simulink model "power_wind_dfig"  (R2023a)
settings: Solver=ode23tb  StartTime=0.0  StopTime=50  MaxStep=1/60  RelTol=1e-4  AbsTol=1e-3  EnableMultiTasking=on
InitFcn:
  | xInitial = init_power_wind_dfig;
undefined symbols (not defined in the file): D1, D11, Delta, F, find_system, Fnom, gcbh, H, ILd_init, ILq_init, Imax_grid_conv, Init, j, Ki_dc_reg, Ki_grid_side_cur_reg, Ki_power_reg, Ki_Q, Ki_rotor_side_cur_reg, Ki_volt_reg, Kp_dc_reg, Kp_grid_side_cur_reg, Kp_power_reg, Kp_Q, Kp_rotor_side_cur_reg, Kp_volt_reg, L_RL, Llr, Lls, p, Pnom, power_A, power_B, power_D, R_RL, Rr, Rs, speed_A, speed_B, speed_C, speed_D, sps_rtmsupport, Vcontrol, Vnom, Wind_On
libraries: spsOnDelayLib x18, spsThreePhaseVIMeasurementLib x6, simulink_extras x5, spsThreePhaseTransformerTwoWindingsLib x4, spsControlledCurrentSourceLib x4, spsGroundLib x3, spsThreePhaseSeriesRLCLoadLib x3, spsPower3phPhasorLib x3, spsBistableLib x3, spsThreePhasePISectionLineLib x2, spsSeriesRLCBranchLib x2, spsSequenceAnalyzerPhasorLib x2
(part 3 of 6)

== system power_wind_dfig/Measurements/Wind turbine Data acquisition/magnitude positive seq. /Fourier1 ==
  signal : Inport
  Constant : Constant  Value=0
  Fcn : Fcn  Expr=u^2
  Fcn1 : Fcn  Expr=u^2
  Fcn2 : Fcn  Expr=sqrt(u)
  Fcn3 : Fcn  Expr=180/pi*atan2(u[2],u[1])
  Gain1 : Gain  Gain=k*f1  SaturateOnIntegerOverflow=on  OutDataTypeStr=Inherit: Same as input  ParamDataTypeStr=Inherit: Same as input
  Integ2 : Integrator  InitialConditionSource=external
  Mux : Mux  Inputs=2
  Product : Product  InputSameDT=on  SaturateOnIntegerOverflow=on  OutDataTypeStr=Inherit: Same as first input
  Product1 : Product  InputSameDT=on  SaturateOnIntegerOverflow=on  OutDataTypeStr=Inherit: Same as first input
  Sum : Sum  InputSameDT=on  SaturateOnIntegerOverflow=on  OutDataTypeStr=Inherit: Same as first input
  Sum1 : Sum  Inputs=+-  InputSameDT=on  SaturateOnIntegerOverflow=on  OutDataTypeStr=Inherit: Same as first input
  Sum2 : Sum  Inputs=+-  InputSameDT=on  SaturateOnIntegerOverflow=on  OutDataTypeStr=Inherit: Same as first input
  T : TransportDelay  DelayTime=1/f1  BufferSize=2048
  T1 : TransportDelay  DelayTime=1/f1  BufferSize=2048
  cos(nwt) : Sin  Frequency=2*pi*n*f1  Phase=pi/2  SampleTime=0
  integ1 : Integrator  InitialConditionSource=external
  sin(nwt) : Sin  Frequency=2*pi*n*f1  SampleTime=0
  magnitude : Outport  InitialOutput=0  VectorParamsAs1DForOutWhenUnconnected=off
  angle : Outport  Port=2  InitialOutput=0  VectorParamsAs1DForOutWhenUnconnected=off
  wires:
  Constant/1 -> integ1/2, Integ2/2
  Sum/1 -> Fcn2/1
  Fcn/1 -> Sum/1
  Fcn1/1 -> Sum/2
  Mux/1 -> Fcn3/1
  Fcn3/1 -> angle/1
  sin(nwt)/1 -> Product/1
  cos(nwt)/1 -> Product1/2
  Product/1 -> integ1/1
  Product1/1 -> Integ2/1
  T/1 -> Sum1/2
  T1/1 -> Sum2/2
  integ1/1 -> Sum1/1, T/1
  Integ2/1 -> T1/1, Sum2/1
  Sum2/1 -> Fcn1/1, Mux/2
  Sum1/1 -> Fcn/1, Mux/1
  signal/1 -> Gain1/1
  Gain1/1 -> Product/2, Product1/1
  Fcn2/1 -> magnitude/1

== system power_wind_dfig/Measurements/Wind turbine Data acquisition/magnitude positive seq. /Fourier2 ==
  signal : Inport
  Constant : Constant  Value=0
  Fcn : Fcn  Expr=u^2
  Fcn1 : Fcn  Expr=u^2
  Fcn2 : Fcn  Expr=sqrt(u)
  Fcn3 : Fcn  Expr=180/pi*atan2(u[2],u[1])
  Gain1 : Gain  Gain=k*f1  SaturateOnIntegerOverflow=on  OutDataTypeStr=Inherit: Same as input  ParamDataTypeStr=Inherit: Same as input
  Integ2 : Integrator  InitialConditionSource=external
  Mux : Mux  Inputs=2
  Product : Product  InputSameDT=on  SaturateOnIntegerOverflow=on  OutDataTypeStr=Inherit: Same as first input
  Product1 : Product  InputSameDT=on  SaturateOnIntegerOverflow=on  OutDataTypeStr=Inherit: Same as first input
  Sum : Sum  InputSameDT=on  SaturateOnIntegerOverflow=on  OutDataTypeStr=Inherit: Same as first input
  Sum1 : Sum  Inputs=+-  InputSameDT=on  SaturateOnIntegerOverflow=on  OutDataTypeStr=Inherit: Same as first input
  Sum2 : Sum  Inputs=+-  InputSameDT=on  SaturateOnIntegerOverflow=on  OutDataTypeStr=Inherit: Same as first input
  T : TransportDelay  DelayTime=1/f1  BufferSize=2048
  T1 : TransportDelay  DelayTime=1/f1  BufferSize=2048
  cos(nwt) : Sin  Frequency=2*pi*n*f1  Phase=pi/2  SampleTime=0
  integ1 : Integrator  InitialConditionSource=external
  sin(nwt) : Sin  Frequency=2*pi*n*f1  SampleTime=0
  magnitude : Outport  InitialOutput=0  VectorParamsAs1DForOutWhenUnconnected=off
  angle : Outport  Port=2  InitialOutput=0  VectorParamsAs1DForOutWhenUnconnected=off
  wires:
  Fcn2/1 -> magnitude/1
  Gain1/1 -> Product1/1, Product/2
  signal/1 -> Gain1/1
  Sum1/1 -> Mux/1, Fcn/1
  Sum2/1 -> Mux/2, Fcn1/1
  Integ2/1 -> Sum2/1, T1/1
  integ1/1 -> T/1, Sum1/1
  T1/1 -> Sum2/2
  T/1 -> Sum1/2
  Product1/1 -> Integ2/1
  Product/1 -> integ1/1
  cos(nwt)/1 -> Product1/2
  sin(nwt)/1 -> Product/1
  Fcn3/1 -> angle/1
  Mux/1 -> Fcn3/1
  Fcn1/1 -> Sum/2
  Fcn/1 -> Sum/1
  Sum/1 -> Fcn2/1
  Constant/1 -> Integ2/2, integ1/2

== system power_wind_dfig/Measurements/Wind turbine Data acquisition/magnitude positivie seq/Fourier1 ==
  signal : Inport
  Constant : Constant  Value=0
  Fcn : Fcn  Expr=u^2
  Fcn1 : Fcn  Expr=u^2
  Fcn2 : Fcn  Expr=sqrt(u)
  Fcn3 : Fcn  Expr=180/pi*atan2(u[2],u[1])
  Gain1 : Gain  Gain=k*f1  SaturateOnIntegerOverflow=on  OutDataTypeStr=Inherit: Same as input  ParamDataTypeStr=Inherit: Same as input
  Integ2 : Integrator  InitialConditionSource=external
  Mux : Mux  Inputs=2
  Product : Product  InputSameDT=on  SaturateOnIntegerOverflow=on  OutDataTypeStr=Inherit: Same as first input
  Product1 : Product  InputSameDT=on  SaturateOnIntegerOverflow=on  OutDataTypeStr=Inherit: Same as first input
  Sum : Sum  InputSameDT=on  SaturateOnIntegerOverflow=on  OutDataTypeStr=Inherit: Same as first input
  Sum1 : Sum  Inputs=+-  InputSameDT=on  SaturateOnIntegerOverflow=on  OutDataTypeStr=Inherit: Same as first input
  Sum2 : Sum  Inputs=+-  InputSameDT=on  SaturateOnIntegerOverflow=on  OutDataTypeStr=Inherit: Same as first input
  T : TransportDelay  DelayTime=1/f1  BufferSize=2048
  T1 : TransportDelay  DelayTime=1/f1  BufferSize=2048
  cos(nwt) : Sin  Frequency=2*pi*n*f1  Phase=pi/2  SampleTime=0
  integ1 : Integrator  InitialConditionSource=external
  sin(nwt) : Sin  Frequency=2*pi*n*f1  SampleTime=0
  magnitude : Outport  InitialOutput=0  VectorParamsAs1DForOutWhenUnconnected=off
  angle : Outport  Port=2  InitialOutput=0  VectorParamsAs1DForOutWhenUnconnected=off
  wires:
  Fcn2/1 -> magnitude/1
  Gain1/1 -> Product1/1, Product/2
  signal/1 -> Gain1/1
  Sum1/1 -> Mux/1, Fcn/1
  Sum2/1 -> Mux/2, Fcn1/1
  Integ2/1 -> Sum2/1, T1/1
  integ1/1 -> T/1, Sum1/1
  T1/1 -> Sum2/2
  T/1 -> Sum1/2
  Product1/1 -> Integ2/1
  Product/1 -> integ1/1
  cos(nwt)/1 -> Product1/2
  sin(nwt)/1 -> Product/1
  Fcn3/1 -> angle/1
  Mux/1 -> Fcn3/1
  Fcn1/1 -> Sum/2
  Fcn/1 -> Sum/1
  Sum/1 -> Fcn2/1
  Constant/1 -> Integ2/2, integ1/2

== system power_wind_dfig/Measurements/Wind turbine Data acquisition/magnitude positivie seq/Fourier2 ==
  signal : Inport
  Constant : Constant  Value=0
  Fcn : Fcn  Expr=u^2
  Fcn1 : Fcn  Expr=u^2
  Fcn2 : Fcn  Expr=sqrt(u)
  Fcn3 : Fcn  Expr=180/pi*atan2(u[2],u[1])
  Gain1 : Gain  Gain=k*f1  SaturateOnIntegerOverflow=on  OutDataTypeStr=Inherit: Same as input  ParamDataTypeStr=Inherit: Same as input
  Integ2 : Integrator  InitialConditionSource=external
  Mux : Mux  Inputs=2
  Product : Product  InputSameDT=on  SaturateOnIntegerOverflow=on  OutDataTypeStr=Inherit: Same as first input
  Product1 : Product  InputSameDT=on  SaturateOnIntegerOverflow=on  OutDataTypeStr=Inherit: Same as first input
  Sum : Sum  InputSameDT=on  SaturateOnIntegerOverflow=on  OutDataTypeStr=Inherit: Same as first input
  Sum1 : Sum  Inputs=+-  InputSameDT=on  SaturateOnIntegerOverflow=on  OutDataTypeStr=Inherit: Same as first input
  Sum2 : Sum  Inputs=+-  InputSameDT=on  SaturateOnIntegerOverflow=on  OutDataTypeStr=Inherit: Same as first input
  T : TransportDelay  DelayTime=1/f1  BufferSize=2048
  T1 : TransportDelay  DelayTime=1/f1  BufferSize=2048
  cos(nwt) : Sin  Frequency=2*pi*n*f1  Phase=pi/2  SampleTime=0
  integ1 : Integrator  InitialConditionSource=external
  sin(nwt) : Sin  Frequency=2*pi*n*f1  SampleTime=0
  magnitude : Outport  InitialOutput=0  VectorParamsAs1DForOutWhenUnconnected=off
  angle : Outport  Port=2  InitialOutput=0  VectorParamsAs1DForOutWhenUnconnected=off
  wires:
  Constant/1 -> integ1/2, Integ2/2
  Sum/1 -> Fcn2/1
  Fcn/1 -> Sum/1
  Fcn1/1 -> Sum/2
  Mux/1 -> Fcn3/1
  Fcn3/1 -> angle/1
  sin(nwt)/1 -> Product/1
  cos(nwt)/1 -> Product1/2
  Product/1 -> integ1/1
  Product1/1 -> Integ2/1
  T/1 -> Sum1/2
  T1/1 -> Sum2/2
  integ1/1 -> Sum1/1, T/1
  Integ2/1 -> T1/1, Sum2/1
  Sum2/1 -> Fcn1/1, Mux/2
  Sum1/1 -> Fcn/1, Mux/1
  signal/1 -> Gain1/1
  Gain1/1 -> Product/2, Product1/1
  Fcn2/1 -> magnitude/1

== system power_wind_dfig/Plant 2 MVA/Plant & Motor Protection/AC Current Protection/Current Measurement ==
  abc : Inport  PortDimensions=3
  Gain1 : Gain  Gain=[1 a a2]  SaturateOnIntegerOverflow=on  OutDataTypeStr=Inherit: Same as input  ParamDataTypeStr=Inherit: Same as input
  Gain2 : Gain  Gain=[1 a2 a]  SaturateOnIntegerOverflow=on  OutDataTypeStr=Inherit: Same as input  ParamDataTypeStr=Inherit: Same as input
  Gain3 : Gain  Gain=1/3  SaturateOnIntegerOverflow=on  OutDataTypeStr=Inherit: Same as input  ParamDataTypeStr=Inherit: Same as input
  Gain4 : Gain  Gain=1/3  SaturateOnIntegerOverflow=on  OutDataTypeStr=Inherit: Same as input  ParamDataTypeStr=Inherit: Same as input
  Mux : Mux  Inputs=3
  Product : Product  Inputs=/*  SaturateOnIntegerOverflow=on  OutDataTypeStr=Inherit: Same as first input
  Saturation : Saturate  UpperLimit=1e6  LowerLimit=1e-6
  Selector : Selector  InputPortWidth=3  IndexOptions=Index vector (dialog)  Indices=1  OutputSizes=1
  Selector1 : Selector  InputPortWidth=3  IndexOptions=Index vector (dialog)  Indices=2  OutputSizes=1
  Selector2 : Selector  InputPortWidth=3  IndexOptions=Index vector (dialog)  Indices=3  OutputSizes=1
  Sum : Sum  Inputs=1  InputSameDT=on  SaturateOnIntegerOverflow=on  OutDataTypeStr=Inherit: Same as first input
  Sum1 : Sum  Inputs=1  InputSameDT=on  SaturateOnIntegerOverflow=on  OutDataTypeStr=Inherit: Same as first input
  magnitude : Subsystem
  magnitude1 : Subsystem
  I1 : Outport  VectorParamsAs1DForOutWhenUnconnected=off
  I2/I1 : Outport  Port=2  VectorParamsAs1DForOutWhenUnconnected=off
  wires:
  magnitude/1(Out1) -> I1/1, Saturation/1
  magnitude1/1(Out1) -> Product/2
  Product/1 -> I2/I1/1
  Saturation/1 -> Product/1
  Gain4/1 -> magnitude1/1(In1)
  Gain3/1 -> magnitude/1(In1)
  Mux/1 -> Gain2/1, Gain1/1
  abc/1 -> Selector/1, Selector1/1, Selector2/1
  Gain2/1 -> Sum1/1
  Sum1/1 -> Gain4/1
  Gain1/1 -> Sum/1
  Sum/1 -> Gain3/1
  Selector/1 -> Mux/1
  Selector1/1 -> Mux/2
  Selector2/1 -> Mux/3

== system power_wind_dfig/Plant 2 MVA/Plant & Motor Protection/AC Voltage Protection/Voltage Measurement ==
  abc : Inport  PortDimensions=3
  Gain1 : Gain  Gain=[1 a a2]  SaturateOnIntegerOverflow=on  OutDataTypeStr=Inherit: Same as input  ParamDataTypeStr=Inherit: Same as input
  Gain2 : Gain  Gain=[1 a2 a]  SaturateOnIntegerOverflow=on  OutDataTypeStr=Inherit: Same as input  ParamDataTypeStr=Inherit: Same as input
  Gain3 : Gain  Gain=1/3  SaturateOnIntegerOverflow=on  OutDataTypeStr=Inherit: Same as input  ParamDataTypeStr=Inherit: Same as input
  Gain4 : Gain  Gain=1/3  SaturateOnIntegerOverflow=on  OutDataTypeStr=Inherit: Same as input  ParamDataTypeStr=Inherit: Same as input
  Gain5 : Gain  Gain=1/3  SaturateOnIntegerOverflow=on  OutDataTypeStr=Inherit: Same as input  ParamDataTypeStr=Inherit: Same as input
  Mux : Mux  Inputs=3
  Product : Product  Inputs=/*  SaturateOnIntegerOverflow=on  OutDataTypeStr=Inherit: Same as first input
  Product1 : Product  Inputs=/*  SaturateOnIntegerOverflow=on  OutDataTypeStr=Inherit: Same as first input
  Saturation : Saturate  UpperLimit=1e6  LowerLimit=1e-6
  Selector : Selector  InputPortWidth=3  IndexOptions=Index vector (dialog)  Indices=1  OutputSizes=1
  Selector1 : Selector  InputPortWidth=3  IndexOptions=Index vector (dialog)  Indices=2  OutputSizes=1
  Selector2 : Selector  InputPortWidth=3  IndexOptions=Index vector (dialog)  Indices=3  OutputSizes=1
  Sum : Sum  Inputs=1  InputSameDT=on  SaturateOnIntegerOverflow=on  OutDataTypeStr=Inherit: Same as first input
  Sum1 : Sum  Inputs=1  InputSameDT=on  SaturateOnIntegerOverflow=on  OutDataTypeStr=Inherit: Same as first input
  Sum2 : Sum  Inputs=1  InputSameDT=on  SaturateOnIntegerOverflow=on  OutDataTypeStr=Inherit: Same as first input
  magnitude : Subsystem
  magnitude1 : Subsystem
  magnitude2 : Subsystem
  V1 : Outport  VectorParamsAs1DForOutWhenUnconnected=off
  V2/V1 : Outport  Port=2  VectorParamsAs1DForOutWhenUnconnected=off
  V0/V1 : Outport  Port=3  VectorParamsAs1DForOutWhenUnconnected=off
  wires:
  magnitude2/1(Out1) -> Product1/2
  magnitude1/1(Out1) -> Product/2
  magnitude/1(Out1) -> Saturation/1, V1/1
  Sum/1 -> Gain3/1
  Gain1/1 -> Sum/1
  Sum1/1 -> Gain4/1
  Gain2/1 -> Sum1/1
  Sum2/1 -> Gain5/1
  Mux/1 -> Gain1/1, Gain2/1, Sum2/1
  Gain3/1 -> magnitude/1(In1)
  Gain4/1 -> magnitude1/1(In1)
  Saturation/1 -> Product/1, Product1/1
  Gain5/1 -> magnitude2/1(In1)
  Product/1 -> V2/V1/1
  Product1/1 -> V0/V1/1
  abc/1 -> Selector/1, Selector1/1, Selector2/1
  Selector/1 -> Mux/1
  Selector1/1 -> Mux/2
  Selector2/1 -> Mux/3

== system power_wind_dfig/Wind Turbine Doubly-Fed Induction Generator (Phasor Type)/Generator & Converters/Asynchronous machine Positive sequence phasor model Inputs and outputs are in per unit (pu)/Mechanical ==
  Tm : Inport
  phiqds1,iqds1 : Inport  Port=2
  1\p : Gain  Gain=1/p  SaturateOnIntegerOverflow=on  OutDataTypeStr=Inherit: Same as input  ParamDataTypeStr=Inherit: Same as input
  1_2H : Gain  Gain=1/(2*H)  SaturateOnIntegerOverflow=on  OutDataTypeStr=Inherit: Same as input  ParamDataTypeStr=Inherit: Same as input
  F : Gain  Gain=F  SaturateOnIntegerOverflow=on  OutDataTypeStr=Inherit: Same as input  ParamDataTypeStr=Inherit: Same as input
  Integrator : Integrator  InitialCondition=wmo  LowerSaturationLimit=0
  Integrator1 : Integrator  InitialCondition=tho
  Mux4 : Mux  Inputs=3
  Product1 : Product  Inputs=1  InputSameDT=on  SaturateOnIntegerOverflow=on  OutDataTypeStr=Inherit: Same as first input
  Product2 : Product  Inputs=1  InputSameDT=on  SaturateOnIntegerOverflow=on  OutDataTypeStr=Inherit: Same as first input
  Selector : Selector  InputPortWidth=4  IndexOptions=Index vector (dialog)  Indices=[1 4]  OutputSizes=1
  Selector1 : Selector  InputPortWidth=4  IndexOptions=Index vector (dialog)  Indices=[2 3]  OutputSizes=1
  Sum : Sum  Inputs=-+-  InputSameDT=on  SaturateOnIntegerOverflow=on  OutDataTypeStr=Inherit: Same as first input
  Sum1 : Sum  Inputs=|-+  InputSameDT=on  SaturateOnIntegerOverflow=on  OutDataTypeStr=Inherit: Same as first input
  web : Gain  Gain=web  SaturateOnIntegerOverflow=on  OutDataTypeStr=Inherit: Same as input  ParamDataTypeStr=Inherit: Same as input
  wr,Te,thr : Outport  VectorParamsAs1DForOutWhenUnconnected=off
  wires:
  Sum1/1 -> Sum/2, Mux4/2  "Pos.seq.Torque"
  Integrator1/1 -> 1\p/1
  1\p/1 -> Mux4/3
  web/1 -> Integrator1/1
  F/1 -> Sum/3
  Integrator/1 -> web/1, Mux4/1, F/1  "w (pu)"
  1_2H/1 -> Integrator/1
  Sum/1 -> 1_2H/1
  Tm/1 -> Sum/1  "Tm"
  Mux4/1 -> wr,Te,thr/1
  Product1/1 -> Sum1/1
  Product2/1 -> Sum1/2
  phiqds1,iqds1/1 -> Selector/1, Selector1/1
  Selector1/1 -> Product2/1
  Selector/1 -> Product1/1

== system power_wind_dfig/Wind Turbine Doubly-Fed Induction Generator (Phasor Type)/Generator & Converters/Asynchronous machine Positive sequence phasor model Inputs and outputs are in per unit (pu)/Phasors Ia Ib stator ==
  note: Ia= I1
  note: Ib= a^2*I1
  note: I1
  Idqs1 : Inport
  Demux : Demux  Outputs=2
      settings: DisplayOption=none
  Mux1 : Mux  Inputs=2
  Mux2 : Mux  Inputs=[2 1]
  Real-Imag to Complex : RealImagToComplex
  Sum : Sum  Inputs=1  InputSameDT=on  SaturateOnIntegerOverflow=on  OutDataTypeStr=Inherit: Same as first input
  a^2 : Gain  Gain=exp(-j*2*pi/3)  SaturateOnIntegerOverflow=on  OutDataTypeStr=Inherit: Same as input  ParamDataTypeStr=Inherit: Same as input
  inv : Gain  Gain=-1  SaturateOnIntegerOverflow=on  OutDataTypeStr=Inherit: Same as input  ParamDataTypeStr=Inherit: Same as input
  Isabc cmplx : Outport  VectorParamsAs1DForOutWhenUnconnected=off
  wires:
  Demux/2 -> Real-Imag to Complex/2
  Demux/1 -> Real-Imag to Complex/1
  a^2/1 -> Mux1/2
  Idqs1/1 -> Demux/1
  Mux1/1 -> Mux2/1, Sum/1  "ia ib"
  Sum/1 -> inv/1
  inv/1 -> Mux2/2  "ic"
  Mux2/1 -> Isabc cmplx/1
  Real-Imag to Complex/1 -> Mux1/1, a^2/1  "I1"

== system power_wind_dfig/Wind Turbine Doubly-Fed Induction Generator (Phasor Type)/Generator & Converters/Asynchronous machine Positive sequence phasor model Inputs and outputs are in per unit (pu)/Positive Sequence Model ==
  Vqdr1 : Inport
  w-wr : Inport  Port=2
  Vqds1 : Inport  Port=3
  Trip : Inport  Port=4
  Constant7 : Constant
  Mutual fluxes : Subsystem
  Rotor : Subsystem
      mask Display: disp('Rotor')
  Stator : Subsystem
      mask Display: disp('Stator')
  Iqdr1 : Outport  VectorParamsAs1DForOutWhenUnconnected=off
  Iqds1 : Outport  Port=2  VectorParamsAs1DForOutWhenUnconnected=off
  Phiqds1_Isqds1 : Outport  Port=3  VectorParamsAs1DForOutWhenUnconnected=off
  wires:
  Stator/3(phis,is) -> Phiqds1_Isqds1/1
  Stator/2(iqs,ids) -> Iqds1/1
  w-wr/1 -> Rotor/2(w-wr)
  Rotor/1(iqr,idr) -> Iqdr1/1
  Vqds1/1 -> Stator/2(vqs,vds)
  Vqdr1/1 -> Rotor/1(vqr,vdr)
  Constant7/1 -> Stator/3(w)
  Rotor/2(phiqr,phidr) -> Mutual fluxes/1(phiqr,phidr)
  Stator/1(phiqs,phids) -> Mutual fluxes/2(phiqs,phids)
  Mutual fluxes/1(phimq,phimd) -> Stator/1(phimq,phimd), Rotor/3(phimq,phimd)
  Trip/1 -> Stator/4(Trip), Rotor/4(Trip)

== system power_wind_dfig/Wind Turbine Doubly-Fed Induction Generator (Phasor Type)/Generator & Converters/Asynchronous machine Positive sequence phasor model Inputs and outputs are in per unit (pu)/Vab Vbc ==
  Vabc : Inport
  Mux : Mux  Inputs=2
  Selector : Selector  InputPortWidth=3  IndexOptions=Index vector (dialog)  Indices=[1]  OutputSizes=1
  Selector1 : Selector  InputPortWidth=3  IndexOptions=Index vector (dialog)  Indices=[2]  OutputSizes=1
  Selector2 : Selector  InputPortWidth=3  IndexOptions=Index vector (dialog)  Indices=[3]  OutputSizes=1
  Sum : Sum  Inputs=|+-  SaturateOnIntegerOverflow=on
  Sum1 : Sum  Inputs=|+-  SaturateOnIntegerOverflow=on
  Vab_Vbc : Outport  VectorParamsAs1DForOutWhenUnconnected=off
  wires:
  Vabc/1 -> Selector2/1, Selector1/1, Selector/1
  Selector/1 -> Sum/1  "Va"
  Selector1/1 -> Sum/2, Sum1/1  "Vb"
  Sum/1 -> Mux/1  "Vab"
  Selector2/1 -> Sum1/2  "Vc"
  Sum1/1 -> Mux/2  "Vbc"
  Mux/1 -> Vab_Vbc/1

== system power_wind_dfig/Wind Turbine Doubly-Fed Induction Generator (Phasor Type)/Generator & Converters/Asynchronous machine Positive sequence phasor model Inputs and outputs are in per unit (pu)/abc2dq ==
  note: V1= 1/3(Vab -a^2*Vbc)
  Vab Vbc cmplx : Inport
  (a^2)/3 : Gain  Gain=1/3*exp(-j*2*pi/3)  SaturateOnIntegerOverflow=on  OutDataTypeStr=Inherit: Same as input  ParamDataTypeStr=Inherit: Same as input
  Complex to Real-Imag : ComplexToRealImag
  Demux : Demux  Outputs=2
      settings: DisplayOption=none
  Gain : Gain  Gain=1/3  SaturateOnIntegerOverflow=on  OutDataTypeStr=Inherit: Same as input  ParamDataTypeStr=Inherit: Same as input
  Mux : Mux  Inputs=2
  Sum3 : Sum  Inputs=+-  InputSameDT=on  SaturateOnIntegerOverflow=on  OutDataTypeStr=Inherit: Same as first input
  Vdqs1 : Outport  VectorParamsAs1DForOutWhenUnconnected=off
  wires:
  Complex to Real-Imag/2 -> Mux/2  "Vq_stator (pu)"
  Complex to Real-Imag/1 -> Mux/1  "Vd_stator (pu)"
  Mux/1 -> Vdqs1/1
  Sum3/1 -> Complex to Real-Imag/1  "V1"
  Demux/1 -> Gain/1
  Vab Vbc cmplx/1 -> Demux/1
  Gain/1 -> Sum3/1
  (a^2)/3/1 -> Sum3/2
  Demux/2 -> (a^2)/3/1

== system power_wind_dfig/Wind Turbine Doubly-Fed Induction Generator (Phasor Type)/Generator & Converters/Control/Converters voltages ==
  Vdq_ctrl_grid_conv : Inport
  Vdc : Inport  Port=2
  Vdq_ctrl_rotor_conv : Inport  Port=3
  ->pu : Gain  Gain=1/(Vnom*sqrt(2)/sqrt(3))  SaturateOnIntegerOverflow=on  OutDataTypeStr=Inherit: Same as input  ParamDataTypeStr=Inherit: Same as input
  "->pu " : Gain  Gain=1/(Vnom*sqrt(2)/sqrt(3))  SaturateOnIntegerOverflow=on  OutDataTypeStr=Inherit: Same as input  ParamDataTypeStr=Inherit: Same as input
  Complex to Real-Imag : ComplexToRealImag
  Complex to Real-Imag1 : ComplexToRealImag
  Gain : Gain  Gain=1/2  SaturateOnIntegerOverflow=on  OutDataTypeStr=Inherit: Same as input  ParamDataTypeStr=Inherit: Same as input
  Gain1 : Gain  Gain=1/2  SaturateOnIntegerOverflow=on  OutDataTypeStr=Inherit: Same as input  ParamDataTypeStr=Inherit: Same as input
  Mux1 : Mux  Inputs=2
  Mux2 : Mux  Inputs=2
  Product1 : Product  Inputs=**  InputSameDT=on  SaturateOnIntegerOverflow=on  OutDataTypeStr=Inherit: Same as first input
  Product2 : Product  Inputs=**  InputSameDT=on  SaturateOnIntegerOverflow=on  OutDataTypeStr=Inherit: Same as first input
  Vdq_grid_conv : Outport  VectorParamsAs1DForOutWhenUnconnected=off
  Vdq_rotor_conv : Outport  Port=2  VectorParamsAs1DForOutWhenUnconnected=off
  wires:
  Vdq_ctrl_rotor_conv/1 -> Product1/2
  Vdq_ctrl_grid_conv/1 -> Product2/1
  Product2/1 -> Gain/1
  Product1/1 -> Gain1/1
  Gain/1 -> ->pu/1
  Gain1/1 -> "->pu "/1
  Vdc/1 -> Product1/1, Product2/2
  ->pu/1 -> Complex to Real-Imag/1
  Complex to Real-Imag1/2 -> Mux2/2  "Vq_rotor (pu)"
  Mux2/1 -> Vdq_rotor_conv/1
  Complex to Real-Imag1/1 -> Mux2/1  "Vd_rotor (pu)"
  "->pu "/1 -> Complex to Real-Imag1/1
  Complex to Real-Imag/1 -> Mux1/1  "Vd_grid_conv (pu)"
  Complex to Real-Imag/2 -> Mux1/2  "Vq_grid_conv (pu)"
  Mux1/1 -> Vdq_grid_conv/1

== system power_wind_dfig/Wind Turbine Doubly-Fed Induction Generator (Phasor Type)/Generator & Converters/Control/abc2dq & Positive sequence Voltage phase angle ==
  note: V1= 1/3(Va +aVb+a^2*Vc)
  Vabc_B1 : Inport
  (a^2)/3 : Gain  Gain=1/3*exp(-j*2*pi/3)  SaturateOnIntegerOverflow=on  OutDataTypeStr=Inherit: Same as input  ParamDataTypeStr=Inherit: Same as input
  20% : Switch  Threshold=0.5  InputSameDT=off
  Complex to Magnitude-Angle : ComplexToMagnitudeAngle
  Complex to Real-Imag : ComplexToRealImag
  Demux : Demux  Outputs=3
      settings: DisplayOption=none
  Gain : Gain  Gain=1/3  SaturateOnIntegerOverflow=on  OutDataTypeStr=Inherit: Same as input  ParamDataTypeStr=Inherit: Same as input
  IC=ic : Memory  InitialCondition=-pi/2  InheritSampleTime=on
  Magnitude-Angle to Complex : MagnitudeAngleToComplex
  Mux : Mux  Inputs=2
  Relay : Relay  OnSwitchValue=0.5  OffSwitchValue=0.1
  Sum3 : Sum  Inputs=+++  InputSameDT=on  SaturateOnIntegerOverflow=on  OutDataTypeStr=Inherit: Same as first input
  a/3 : Gain  Gain=1/3*exp(j*2*pi/3)  SaturateOnIntegerOverflow=on  OutDataTypeStr=Inherit: Same as input  ParamDataTypeStr=Inherit: Same as input
  Vdq_B1 : Outport  VectorParamsAs1DForOutWhenUnconnected=off
  Theta : Outport  Port=2  VectorParamsAs1DForOutWhenUnconnected=off
  V_B1 : Outport  Port=3  VectorParamsAs1DForOutWhenUnconnected=off
  wires:
  Complex to Real-Imag/2 -> Mux/2  "Vq"
  Complex to Real-Imag/1 -> Mux/1  "Vd"
  Magnitude-Angle to Complex/1 -> Complex to Real-Imag/1
  Complex to Magnitude-Angle/1 -> Relay/1, Magnitude-Angle to Complex/1, V_B1/1
  Sum3/1 -> Complex to Magnitude-Angle/1  "V1"
  (a^2)/3/1 -> Sum3/3
  a/3/1 -> Sum3/2
  Demux/3 -> (a^2)/3/1
  Demux/2 -> a/3/1
  Gain/1 -> Sum3/1
  Vabc_B1/1 -> Demux/1
  Demux/1 -> Gain/1
  Mux/1 -> Vdq_B1/1
  20%/1 -> Theta/1, IC=ic/1
  IC=ic/1 -> 20%/3
  Relay/1 -> 20%/2
  Complex to Magnitude-Angle/2 -> Magnitude-Angle to Complex/2, 20%/1

== system power_wind_dfig/Wind Turbine Doubly-Fed Induction Generator (Phasor Type)/Generator & Converters/Control/wind_dfig_grid ==
  note: Grid-side converter control system
  Vdq_B1 : Inport
  Idq_grid_conv : Inport  Port=2
  Theta : Inport  Port=3
  Vdc : Inport  Port=4
  Iq_ref : Inport  Port=5
  Enable : EnablePort  PropagateVarSize=During execution
  Current regulator : Subsystem
  DC bus voltage Regulator : Subsystem
  Idq B1 voltage Reference frame : Subsystem
  Idq references : Subsystem
  Mux : Mux  Inputs=2
  Rate Limiter : RateLimiter  RisingSlewLimit=current_slew_rate  FallingSlewLimit=-current_slew_rate
  Subsystem : Subsystem
  Vdc_ref (V) : Constant  Value=Vdc_nom
  Vdq B1 voltage Reference frame : Subsystem
  Vdq_ctrl_grid_conv : Outport  VectorParamsAs1DForOutWhenUnconnected=off
  wires:
  Iq_ref/1 -> Rate Limiter/1
  Rate Limiter/1 -> Mux/2
  Idq references/1(Idq_ref) -> Current regulator/3(Idq_ref)
  Mux/1 -> Idq references/1(Id*Iq*)
  Idq B1 voltage Reference frame/1(Idq) -> Current regulator/2(Idq)
  DC bus voltage Regulator/1(Id_ref) -> Mux/1
  Idq_grid_conv/1 -> Idq B1 voltage Reference frame/2(Idq_grid_conv)
  Subsystem/1(Vdq_ctrl_grid_conv) -> Vdq_ctrl_grid_conv/1
  Vdc/1 -> DC bus voltage Regulator/2(Vdc), Subsystem/3(Vdc)
  Current regulator/1(Vdq*) -> Subsystem/2(Vdq*)
  Vdc_ref (V)/1 -> DC bus voltage Regulator/1(Vdc_ref)
  Theta/1 -> Subsystem/1(Theta), Vdq B1 voltage Reference frame/1(Theta), Idq B1 voltage Reference frame/1(Theta)
  Vdq_B1/1 -> Vdq B1 voltage Reference frame/2(Vdq_B1)
  Vdq B1 voltage Reference frame/1(Vdq) -> Current regulator/1(Vdq)

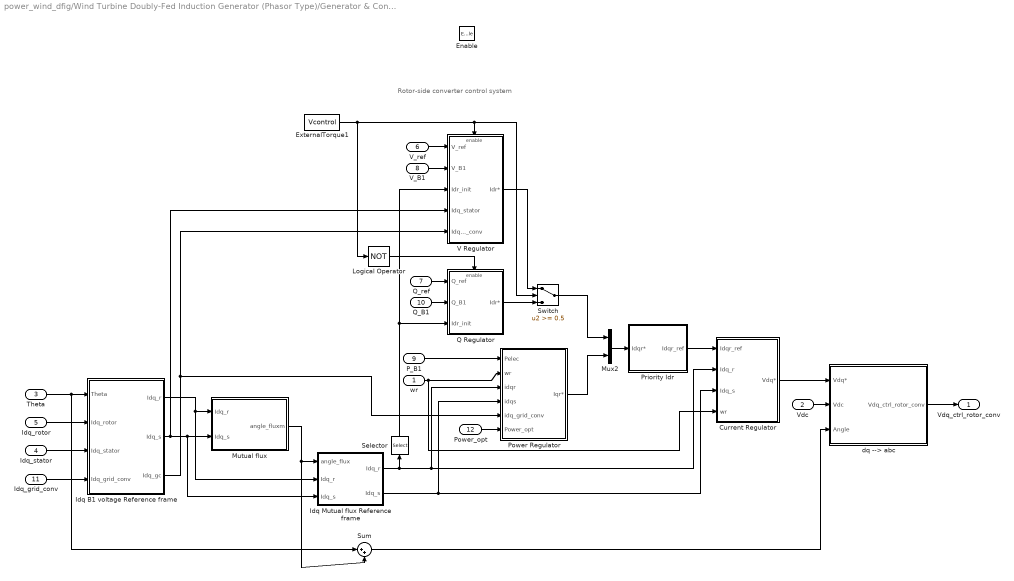
== system power_wind_dfig/Wind Turbine Doubly-Fed Induction Generator (Phasor Type)/Generator & Converters/Control/wind_dfig_rotor ==
  note: Rotor-side converter control system
  wr : Inport
  Vdc : Inport  Port=2
  Theta : Inport  Port=3
  Idq_stator : Inport  Port=4
  Idq_rotor : Inport  Port=5
  V_ref : Inport  Port=6
  Q_ref : Inport  Port=7
  V_B1 : Inport  Port=8
  P_B1 : Inport  Port=9
  Q_B1 : Inport  Port=10
  Idq_grid_conv : Inport  Port=11
  Power_opt : Inport  Port=12
  Enable : EnablePort  PropagateVarSize=During execution
  Current Regulator : Subsystem
  ExternalTorque1 : Constant  Value=Vcontrol
  Idq B1 voltage Reference frame : Subsystem
  Idq Mutual flux Reference frame : Subsystem
  Logical Operator : Logic  Operator=NOT  AllPortsSameDT=off
  Mutual flux : Subsystem
  Mux2 : Mux  Inputs=2
  Power Regulator : Subsystem
  Priority Idr : Subsystem
  Q Regulator : Subsystem
  Selector : Selector  InputPortWidth=2  IndexOptions=Index vector (dialog)  Indices=1  OutputSizes=1
  Sum : Sum  Inputs=|++  SaturateOnIntegerOverflow=on
  Switch : Switch  Threshold=0.5  InputSameDT=off
  V Regulator : Subsystem
  dq --> abc : Subsystem
  Vdq_ctrl_rotor_conv : Outport  VectorParamsAs1DForOutWhenUnconnected=off
  wires:
  Mutual flux/1(angle_fluxm) -> Sum/2, Idq Mutual flux Reference frame/1(angle_flux)
  wr/1 -> Current Regulator/4(wr), Power Regulator/2(wr)
  Mux2/1 -> Priority Idr/1(Idqr*)
  Current Regulator/1(Vdq*) -> dq --> abc/1(Vdq*)
  Vdc/1 -> dq --> abc/2(Vdc)
  Theta/1 -> Sum/1, Idq B1 voltage Reference frame/1(Theta)
  Idq Mutual flux Reference frame/1("Idq_r ") -> Selector/1, Current Regulator/2(Idq_r), Power Regulator/3(idqr)
  Sum/1 -> dq --> abc/3(Angle)
  dq --> abc/1(Vdq_ctrl_rotor_conv) -> Vdq_ctrl_rotor_conv/1
  Idq B1 voltage Reference frame/2(Idq_s) -> Idq Mutual flux Reference frame/3(Idq_s), Mutual flux/2(Idq_s), V Regulator/4(Idq_stator)
  Idq Mutual flux Reference frame/2("Idq_s ") -> Current Regulator/3(Idq_s), Power Regulator/4(idqs)
  Idq_rotor/1 -> Idq B1 voltage Reference frame/2(Idq_rotor)
  Idq_stator/1 -> Idq B1 voltage Reference frame/3(Idq_stator)
  Idq B1 voltage Reference frame/1(Idq_r) -> Mutual flux/1(Idq_r), Idq Mutual flux Reference frame/2(Idq_r)
  Q_ref/1 -> Q Regulator/1(Q_ref)
  Q_B1/1 -> Q Regulator/2(Q_B1)
  Selector/1 -> V Regulator/3(Idr_init), Q Regulator/3(Idr_init)
  P_B1/1 -> Power Regulator/1(Pelec)
  V_ref/1 -> V Regulator/1(V_ref)
  V_B1/1 -> V Regulator/2(V_B1)
  ExternalTorque1/1 -> Logical Operator/1, Switch/2, V Regulator/Enable
  Logical Operator/1 -> Q Regulator/Enable
  Q Regulator/1(Idr*) -> Switch/3
  V Regulator/1(Idr*) -> Switch/1
  Idq B1 voltage Reference frame/3(Idq_gc) -> V Regulator/5(Idq_grid_conv), Power Regulator/5(idq_grid_conv)
  Idq_grid_conv/1 -> Idq B1 voltage Reference frame/4(Idq_grid_conv)
  Priority Idr/1(Idqr_ref) -> Current Regulator/1(Idqr_ref)
  Power_opt/1 -> Power Regulator/6(Power_opt)
  Switch/1 -> Mux2/1
  Power Regulator/1(Iqr*) -> Mux2/2

== system power_wind_dfig/Wind Turbine Doubly-Fed Induction Generator (Phasor Type)/Generator & Converters/Grid-side converter currents & Converters power/d-q axis model of a 3-phase series R-L branch ==
  note: where w = 2*pi*Fnom (Hz)
  note: Vq1 - Vq2 = [ R * Iq ] + [ L* w * Id ] + [ L * d/dt (Iq) ]
  note: ==========================================================================================
  note: I --->
  note: V2
  note: V1
  note: o--------| R |---| L |-------o
  note: Vd1 - Vd2 = [ R * Id ] - [ L* w * Iq ] + [ L * d/dt (Id) ]
  note: where w = 2*pi*Fnom (Hz)
  note: Iq = [ w / ( L * s ) ] * [ Vq1 - Vq2 - ( R * Iq ) - ( L * Id ) ]
  note: Id = [ w / ( L * s ) ] * [ Vd1 - Vd2 - ( R * Id ) + ( L * Iq ) ]
  note: d-q axis model of a 3-phase series R-L branch
  note: Using Laplace transform and per unit (pu) quantities :
  Vdq1 : Inport
  Vdq2 : Inport  Port=2
  Trip : Inport  Port=3
  Constant : Constant  Value=0
  Integrator : Integrator  InitialCondition=Idq0
  R_choke : Gain  Gain=R  SaturateOnIntegerOverflow=on  OutDataTypeStr=Inherit: Same as input  ParamDataTypeStr=Inherit: Same as input
  R_choke1 : Gain  Gain=L  SaturateOnIntegerOverflow=on  OutDataTypeStr=Inherit: Same as input  ParamDataTypeStr=Inherit: Same as input
  R_choke2 : Gain  Gain=[1 -1]  SaturateOnIntegerOverflow=on  OutDataTypeStr=Inherit: Same as input  ParamDataTypeStr=Inherit: Same as input
  R_choke3 : Gain  Gain=w / L  SaturateOnIntegerOverflow=on  OutDataTypeStr=Inherit: Same as input  ParamDataTypeStr=Inherit: Same as input
  Selector : Selector  InputPortWidth=2  IndexOptions=Index vector (dialog)  Indices=[2 1]  OutputSizes=1
  Sum : Sum  Inputs=+--+  SaturateOnIntegerOverflow=on
  Switch : Switch  Criteria=u2 ~= 0  Threshold=0.5  InputSameDT=off
  Switch1 : Switch  Criteria=u2 ~= 0  Threshold=0.5  InputSameDT=off
  Idq : Outport  VectorParamsAs1DForOutWhenUnconnected=off
  wires:
  Selector/1 -> R_choke1/1
  Sum/1 -> R_choke3/1
  R_choke1/1 -> R_choke2/1
  R_choke2/1 -> Sum/4
  R_choke/1 -> Sum/3
  Vdq2/1 -> Sum/2
  Vdq1/1 -> Sum/1
  Switch/1 -> Integrator/1
  R_choke3/1 -> Switch/3
  Constant/1 -> Switch/1, Switch1/1
  Switch1/1 -> Idq/1, Selector/1, R_choke/1
  Integrator/1 -> Switch1/3
  Trip/1 -> Switch/2, Switch1/2

== system power_wind_dfig/Wind Turbine Doubly-Fed Induction Generator (Phasor Type)/Generator & Converters/Grid-side converter currents & Converters power/dq2ab ==
  note: Ia = I1
      | Ib = (a^2 * I1)
  Idq_seq1 : Inport
  Demux1 : Demux  Outputs=2
      settings: DisplayOption=none
  Mux : Mux  Inputs=2
  Real-Imag to Complex1 : RealImagToComplex
  a^2 : Gain  Gain=exp(-j*2*pi/3)  SaturateOnIntegerOverflow=on  OutDataTypeStr=Inherit: Same as input  ParamDataTypeStr=Inherit: Same as input
  Ia_Ib complx : Outport  VectorParamsAs1DForOutWhenUnconnected=off
  wires:
  Mux/1 -> Ia_Ib complx/1
  Idq_seq1/1 -> Demux1/1
  Demux1/1 -> Real-Imag to Complex1/1
  Demux1/2 -> Real-Imag to Complex1/2
  Real-Imag to Complex1/1 -> Mux/1, a^2/1  "I1"
  a^2/1 -> Mux/2

== system power_wind_dfig/Wind Turbine Protection/Protection System/AC Current Protection/Current Measurement ==
  abc : Inport  PortDimensions=3
  Gain1 : Gain  Gain=[1 a a2]  SaturateOnIntegerOverflow=on  OutDataTypeStr=Inherit: Same as input  ParamDataTypeStr=Inherit: Same as input
  Gain2 : Gain  Gain=[1 a2 a]  SaturateOnIntegerOverflow=on  OutDataTypeStr=Inherit: Same as input  ParamDataTypeStr=Inherit: Same as input
  Gain3 : Gain  Gain=1/3  SaturateOnIntegerOverflow=on  OutDataTypeStr=Inherit: Same as input  ParamDataTypeStr=Inherit: Same as input
  Gain4 : Gain  Gain=1/3  SaturateOnIntegerOverflow=on  OutDataTypeStr=Inherit: Same as input  ParamDataTypeStr=Inherit: Same as input
  Mux : Mux  Inputs=3
  Product : Product  Inputs=/*  SaturateOnIntegerOverflow=on  OutDataTypeStr=Inherit: Same as first input
  Saturation : Saturate  UpperLimit=1e6  LowerLimit=1e-6
  Selector : Selector  InputPortWidth=3  IndexOptions=Index vector (dialog)  Indices=1  OutputSizes=1
  Selector1 : Selector  InputPortWidth=3  IndexOptions=Index vector (dialog)  Indices=2  OutputSizes=1
  Selector2 : Selector  InputPortWidth=3  IndexOptions=Index vector (dialog)  Indices=3  OutputSizes=1
  Sum : Sum  Inputs=1  InputSameDT=on  SaturateOnIntegerOverflow=on  OutDataTypeStr=Inherit: Same as first input
  Sum1 : Sum  Inputs=1  InputSameDT=on  SaturateOnIntegerOverflow=on  OutDataTypeStr=Inherit: Same as first input
  magnitude : Subsystem
  magnitude1 : Subsystem
  I1 : Outport  VectorParamsAs1DForOutWhenUnconnected=off
  I2/I1 : Outport  Port=2  VectorParamsAs1DForOutWhenUnconnected=off
  wires:
  Selector2/1 -> Mux/3
  Selector1/1 -> Mux/2
  Selector/1 -> Mux/1
  Sum/1 -> Gain3/1
  Gain1/1 -> Sum/1
  Sum1/1 -> Gain4/1
  Gain2/1 -> Sum1/1
  abc/1 -> Selector2/1, Selector1/1, Selector/1
  Mux/1 -> Gain1/1, Gain2/1
  Gain3/1 -> magnitude/1(In1)
  Gain4/1 -> magnitude1/1(In1)
  Saturation/1 -> Product/1
  Product/1 -> I2/I1/1
  magnitude1/1(Out1) -> Product/2
  magnitude/1(Out1) -> Saturation/1, I1/1

== system power_wind_dfig/Wind Turbine Protection/Protection System/AC Voltage Protection/Voltage Measurement ==
  abc : Inport  PortDimensions=3
  Gain1 : Gain  Gain=[1 a a2]  SaturateOnIntegerOverflow=on  OutDataTypeStr=Inherit: Same as input  ParamDataTypeStr=Inherit: Same as input
  Gain2 : Gain  Gain=[1 a2 a]  SaturateOnIntegerOverflow=on  OutDataTypeStr=Inherit: Same as input  ParamDataTypeStr=Inherit: Same as input
  Gain3 : Gain  Gain=1/3  SaturateOnIntegerOverflow=on  OutDataTypeStr=Inherit: Same as input  ParamDataTypeStr=Inherit: Same as input
  Gain4 : Gain  Gain=1/3  SaturateOnIntegerOverflow=on  OutDataTypeStr=Inherit: Same as input  ParamDataTypeStr=Inherit: Same as input
  Gain5 : Gain  Gain=1/3  SaturateOnIntegerOverflow=on  OutDataTypeStr=Inherit: Same as input  ParamDataTypeStr=Inherit: Same as input
  Mux : Mux  Inputs=3
  Product : Product  Inputs=/*  SaturateOnIntegerOverflow=on  OutDataTypeStr=Inherit: Same as first input
  Product1 : Product  Inputs=/*  SaturateOnIntegerOverflow=on  OutDataTypeStr=Inherit: Same as first input
  Saturation : Saturate  UpperLimit=1e6  LowerLimit=1e-6
  Selector : Selector  InputPortWidth=3  IndexOptions=Index vector (dialog)  Indices=1  OutputSizes=1
  Selector1 : Selector  InputPortWidth=3  IndexOptions=Index vector (dialog)  Indices=2  OutputSizes=1
  Selector2 : Selector  InputPortWidth=3  IndexOptions=Index vector (dialog)  Indices=3  OutputSizes=1
  Sum : Sum  Inputs=1  InputSameDT=on  SaturateOnIntegerOverflow=on  OutDataTypeStr=Inherit: Same as first input
  Sum1 : Sum  Inputs=1  InputSameDT=on  SaturateOnIntegerOverflow=on  OutDataTypeStr=Inherit: Same as first input
  Sum2 : Sum  Inputs=1  InputSameDT=on  SaturateOnIntegerOverflow=on  OutDataTypeStr=Inherit: Same as first input
  magnitude : Subsystem
  magnitude1 : Subsystem
  magnitude2 : Subsystem
  V1 : Outport  VectorParamsAs1DForOutWhenUnconnected=off
  V2/V1 : Outport  Port=2  VectorParamsAs1DForOutWhenUnconnected=off
  V0/V1 : Outport  Port=3  VectorParamsAs1DForOutWhenUnconnected=off
  wires:
  Selector2/1 -> Mux/3
  Selector1/1 -> Mux/2
  Selector/1 -> Mux/1
  abc/1 -> Selector2/1, Selector1/1, Selector/1
  Product1/1 -> V0/V1/1
  Product/1 -> V2/V1/1
  Gain5/1 -> magnitude2/1(In1)
  Saturation/1 -> Product1/1, Product/1
  Gain4/1 -> magnitude1/1(In1)
  Gain3/1 -> magnitude/1(In1)
  Mux/1 -> Sum2/1, Gain2/1, Gain1/1
  Sum2/1 -> Gain5/1
  Gain2/1 -> Sum1/1
  Sum1/1 -> Gain4/1
  Gain1/1 -> Sum/1
  Sum/1 -> Gain3/1
  magnitude/1(Out1) -> V1/1, Saturation/1
  magnitude1/1(Out1) -> Product/2
  magnitude2/1(Out1) -> Product1/2

== system power_wind_dfig/Plant 2 MVA/Plant & Motor Protection/AC Current Protection/Current Measurement/magnitude ==
  In1 : Inport
  Complex to Real-Imag : ComplexToRealImag
  Fourier1 : Subsystem  mask(Fourier analyser){f1=Freq, n=0}
      mask prompts: f1 "Fundamental frequency f1 (Hz):"; n "Harmonic n (0=DC; 1=fundamental; 2=2nd harm;  ...) :"
      mask help: The Fourier block performs a Fourier analysis of the input signal over a running window of one cycle of the fundamental frequency. First and second outputs return respectively the magnitude and phase (degrees) of the harmonic component specified.
      mask init:
      | k=2-(n==0);
      mask Help: helpview(psbhelp)
  Fourier2 : Subsystem  mask(Fourier analyser){f1=Freq, n=0}
      mask prompts: f1 "Fundamental frequency f1 (Hz):"; n "Harmonic n (0=DC; 1=fundamental; 2=2nd harm;  ...) :"
      mask help: The Fourier block performs a Fourier analysis of the input signal over a running window of one cycle of the fundamental frequency. First and second outputs return respectively the magnitude and phase (degrees) of the harmonic component specified.
      mask init:
      | k=2-(n==0);
      mask Help: helpview(psbhelp)
  Math Function : Math  Operator=hypot  SignedPower=on
  Terminator : Terminator
  Terminator1 : Terminator
  Out1 : Outport  VectorParamsAs1DForOutWhenUnconnected=off
  wires:
  In1/1 -> Complex to Real-Imag/1
  Math Function/1 -> Out1/1
  Fourier2/1(magnitude) -> Math Function/2
  Fourier1/1(magnitude) -> Math Function/1
  Fourier2/2(angle) -> Terminator1/1
  Fourier1/2(angle) -> Terminator/1
  Complex to Real-Imag/2 -> Fourier2/1(signal)
  Complex to Real-Imag/1 -> Fourier1/1(signal)

== system power_wind_dfig/Plant 2 MVA/Plant & Motor Protection/AC Current Protection/Current Measurement/magnitude1 ==
  In1 : Inport
  Complex to Real-Imag : ComplexToRealImag
  Fourier1 : Subsystem  mask(Fourier analyser){f1=Freq, n=0}
      mask prompts: f1 "Fundamental frequency f1 (Hz):"; n "Harmonic n (0=DC; 1=fundamental; 2=2nd harm;  ...) :"
      mask help: The Fourier block performs a Fourier analysis of the input signal over a running window of one cycle of the fundamental frequency. First and second outputs return respectively the magnitude and phase (degrees) of the harmonic component specified.
      mask init:
      | k=2-(n==0);
      mask Help: helpview(psbhelp)
  Fourier2 : Subsystem  mask(Fourier analyser){f1=Freq, n=0}
      mask prompts: f1 "Fundamental frequency f1 (Hz):"; n "Harmonic n (0=DC; 1=fundamental; 2=2nd harm;  ...) :"
      mask help: The Fourier block performs a Fourier analysis of the input signal over a running window of one cycle of the fundamental frequency. First and second outputs return respectively the magnitude and phase (degrees) of the harmonic component specified.
      mask init:
      | k=2-(n==0);
      mask Help: helpview(psbhelp)
  Math Function : Math  Operator=hypot  SignedPower=on
  Terminator : Terminator
  Terminator1 : Terminator
  Out1 : Outport  VectorParamsAs1DForOutWhenUnconnected=off
  wires:
  Complex to Real-Imag/1 -> Fourier1/1(signal)
  Complex to Real-Imag/2 -> Fourier2/1(signal)
  Fourier1/2(angle) -> Terminator/1
  Fourier2/2(angle) -> Terminator1/1
  Fourier1/1(magnitude) -> Math Function/1
  Fourier2/1(magnitude) -> Math Function/2
  Math Function/1 -> Out1/1
  In1/1 -> Complex to Real-Imag/1

== system power_wind_dfig/Plant 2 MVA/Plant & Motor Protection/AC Voltage Protection/Voltage Measurement/magnitude ==
  In1 : Inport
  Complex to Real-Imag : ComplexToRealImag
  Fourier1 : Subsystem  mask(Fourier analyser){f1=Freq, n=0}
      mask prompts: f1 "Fundamental frequency f1 (Hz):"; n "Harmonic n (0=DC; 1=fundamental; 2=2nd harm;  ...) :"
      mask help: The Fourier block performs a Fourier analysis of the input signal over a running window of one cycle of the fundamental frequency. First and second outputs return respectively the magnitude and phase (degrees) of the harmonic component specified.
      mask init:
      | k=2-(n==0);
      mask Help: helpview(psbhelp)
  Fourier2 : Subsystem  mask(Fourier analyser){f1=Freq, n=0}
      mask prompts: f1 "Fundamental frequency f1 (Hz):"; n "Harmonic n (0=DC; 1=fundamental; 2=2nd harm;  ...) :"
      mask help: The Fourier block performs a Fourier analysis of the input signal over a running window of one cycle of the fundamental frequency. First and second outputs return respectively the magnitude and phase (degrees) of the harmonic component specified.
      mask init:
      | k=2-(n==0);
      mask Help: helpview(psbhelp)
  Math Function : Math  Operator=hypot  SignedPower=on
  Terminator : Terminator
  Terminator1 : Terminator
  Out1 : Outport  VectorParamsAs1DForOutWhenUnconnected=off
  wires:
  In1/1 -> Complex to Real-Imag/1
  Math Function/1 -> Out1/1
  Fourier2/1(magnitude) -> Math Function/2
  Fourier1/1(magnitude) -> Math Function/1
  Fourier2/2(angle) -> Terminator1/1
  Fourier1/2(angle) -> Terminator/1
  Complex to Real-Imag/2 -> Fourier2/1(signal)
  Complex to Real-Imag/1 -> Fourier1/1(signal)

== system power_wind_dfig/Plant 2 MVA/Plant & Motor Protection/AC Voltage Protection/Voltage Measurement/magnitude1 ==
  In1 : Inport
  Complex to Real-Imag : ComplexToRealImag
  Fourier1 : Subsystem  mask(Fourier analyser){f1=Freq, n=0}
      mask prompts: f1 "Fundamental frequency f1 (Hz):"; n "Harmonic n (0=DC; 1=fundamental; 2=2nd harm;  ...) :"
      mask help: The Fourier block performs a Fourier analysis of the input signal over a running window of one cycle of the fundamental frequency. First and second outputs return respectively the magnitude and phase (degrees) of the harmonic component specified.
      mask init:
      | k=2-(n==0);
      mask Help: helpview(psbhelp)
  Fourier2 : Subsystem  mask(Fourier analyser){f1=Freq, n=0}
      mask prompts: f1 "Fundamental frequency f1 (Hz):"; n "Harmonic n (0=DC; 1=fundamental; 2=2nd harm;  ...) :"
      mask help: The Fourier block performs a Fourier analysis of the input signal over a running window of one cycle of the fundamental frequency. First and second outputs return respectively the magnitude and phase (degrees) of the harmonic component specified.
      mask init:
      | k=2-(n==0);
      mask Help: helpview(psbhelp)
  Math Function : Math  Operator=hypot  SignedPower=on
  Terminator : Terminator
  Terminator1 : Terminator
  Out1 : Outport  VectorParamsAs1DForOutWhenUnconnected=off
  wires:
  Complex to Real-Imag/1 -> Fourier1/1(signal)
  Complex to Real-Imag/2 -> Fourier2/1(signal)
  Fourier1/2(angle) -> Terminator/1
  Fourier2/2(angle) -> Terminator1/1
  Fourier1/1(magnitude) -> Math Function/1
  Fourier2/1(magnitude) -> Math Function/2
  Math Function/1 -> Out1/1
  In1/1 -> Complex to Real-Imag/1

== system power_wind_dfig/Plant 2 MVA/Plant & Motor Protection/AC Voltage Protection/Voltage Measurement/magnitude2 ==
  In1 : Inport
  Complex to Real-Imag : ComplexToRealImag
  Fourier1 : Subsystem  mask(Fourier analyser){f1=Freq, n=0}
      mask prompts: f1 "Fundamental frequency f1 (Hz):"; n "Harmonic n (0=DC; 1=fundamental; 2=2nd harm;  ...) :"
      mask help: The Fourier block performs a Fourier analysis of the input signal over a running window of one cycle of the fundamental frequency. First and second outputs return respectively the magnitude and phase (degrees) of the harmonic component specified.
      mask init:
      | k=2-(n==0);
      mask Help: helpview(psbhelp)
  Fourier2 : Subsystem  mask(Fourier analyser){f1=Freq, n=0}
      mask prompts: f1 "Fundamental frequency f1 (Hz):"; n "Harmonic n (0=DC; 1=fundamental; 2=2nd harm;  ...) :"
      mask help: The Fourier block performs a Fourier analysis of the input signal over a running window of one cycle of the fundamental frequency. First and second outputs return respectively the magnitude and phase (degrees) of the harmonic component specified.
      mask init:
      | k=2-(n==0);
      mask Help: helpview(psbhelp)
  Math Function : Math  Operator=hypot  SignedPower=on
  Terminator : Terminator
  Terminator1 : Terminator
  Out1 : Outport  VectorParamsAs1DForOutWhenUnconnected=off
  wires:
  In1/1 -> Complex to Real-Imag/1
  Math Function/1 -> Out1/1
  Fourier2/1(magnitude) -> Math Function/2
  Fourier1/1(magnitude) -> Math Function/1
  Fourier2/2(angle) -> Terminator1/1
  Fourier1/2(angle) -> Terminator/1
  Complex to Real-Imag/2 -> Fourier2/1(signal)
  Complex to Real-Imag/1 -> Fourier1/1(signal)

== system power_wind_dfig/Wind Turbine Doubly-Fed Induction Generator (Phasor Type)/Generator & Converters/Asynchronous machine Positive sequence phasor model Inputs and outputs are in per unit (pu)/Positive Sequence Model/Mutual fluxes ==
  phiqr,phidr : Inport
  phiqs,phids : Inport  Port=2
  1\Llr : Gain  Gain=1/Llr  SaturateOnIntegerOverflow=on  OutDataTypeStr=Inherit: Same as input  ParamDataTypeStr=Inherit: Same as input
  1\Llr1 : Gain  Gain=Laq  SaturateOnIntegerOverflow=on  OutDataTypeStr=Inherit: Same as input  ParamDataTypeStr=Inherit: Same as input
  1\Llr2 : Gain  Gain=Lad  SaturateOnIntegerOverflow=on  OutDataTypeStr=Inherit: Same as input  ParamDataTypeStr=Inherit: Same as input
  1\Lls : Gain  Gain=1/Lls  SaturateOnIntegerOverflow=on  OutDataTypeStr=Inherit: Same as input  ParamDataTypeStr=Inherit: Same as input
  Demux1 : Demux  Outputs=2
      settings: DisplayOption=none
  Demux2 : Demux  Outputs=2
      settings: DisplayOption=none
  Mux3 : Mux  Inputs=2
  Sum : Sum  Inputs=|++  InputSameDT=on  SaturateOnIntegerOverflow=on  OutDataTypeStr=Inherit: Same as first input
  Sum1 : Sum  Inputs=++|  InputSameDT=on  SaturateOnIntegerOverflow=on  OutDataTypeStr=Inherit: Same as first input
  phimq,phimd : Outport  VectorParamsAs1DForOutWhenUnconnected=off
  wires:
  Mux3/1 -> phimq,phimd/1
  1\Llr2/1 -> Mux3/2
  1\Llr1/1 -> Mux3/1
  Demux1/2 -> Sum1/1
  Demux2/2 -> Sum1/2
  Demux2/1 -> Sum/2
  1\Lls/1 -> Demux2/1
  Sum/1 -> 1\Llr1/1
  1\Llr/1 -> Demux1/1
  phiqr,phidr/1 -> 1\Llr/1
  phiqs,phids/1 -> 1\Lls/1
  Sum1/1 -> 1\Llr2/1
  Demux1/1 -> Sum/1

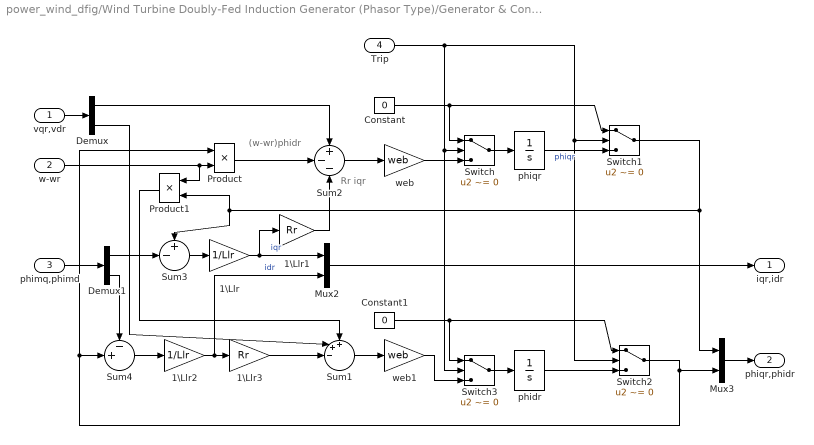
== system power_wind_dfig/Wind Turbine Doubly-Fed Induction Generator (Phasor Type)/Generator & Converters/Asynchronous machine Positive sequence phasor model Inputs and outputs are in per unit (pu)/Positive Sequence Model/Rotor ==
  note: Rr iqr
  note: (w-wr)phidr
  vqr,vdr : Inport
  w-wr : Inport  Port=2
  phimq,phimd : Inport  Port=3
  Trip : Inport  Port=4
  1\Llr : Gain  Gain=1/Llr  SaturateOnIntegerOverflow=on  OutDataTypeStr=Inherit: Same as input  ParamDataTypeStr=Inherit: Same as input
  1\Llr1 : Gain  Gain=Rr  SaturateOnIntegerOverflow=on  OutDataTypeStr=Inherit: Same as input  ParamDataTypeStr=Inherit: Same as input
  1\Llr2 : Gain  Gain=1/Llr  SaturateOnIntegerOverflow=on  OutDataTypeStr=Inherit: Same as input  ParamDataTypeStr=Inherit: Same as input
  1\Llr3 : Gain  Gain=Rr  SaturateOnIntegerOverflow=on  OutDataTypeStr=Inherit: Same as input  ParamDataTypeStr=Inherit: Same as input
  Constant : Constant  Value=0
  Constant1 : Constant  Value=0
  Demux : Demux  Outputs=2
      settings: DisplayOption=none
  Demux1 : Demux  Outputs=2
      settings: DisplayOption=none
  Mux2 : Mux  Inputs=2
  Mux3 : Mux  Inputs=2
  Product : Product  InputSameDT=on  SaturateOnIntegerOverflow=on  OutDataTypeStr=Inherit: Same as first input
  Product1 : Product  InputSameDT=on  SaturateOnIntegerOverflow=on  OutDataTypeStr=Inherit: Same as first input
  Sum1 : Sum  Inputs=++-||  InputSameDT=on  SaturateOnIntegerOverflow=on  OutDataTypeStr=Inherit: Same as first input
  Sum2 : Sum  Inputs=+--  InputSameDT=on  SaturateOnIntegerOverflow=on  OutDataTypeStr=Inherit: Same as first input
  Sum3 : Sum  Inputs=+-|  InputSameDT=on  SaturateOnIntegerOverflow=on  OutDataTypeStr=Inherit: Same as first input
  Sum4 : Sum  Inputs=-+|  InputSameDT=on  SaturateOnIntegerOverflow=on  OutDataTypeStr=Inherit: Same as first input
  Switch{,1..3} (4 alike) : Switch  Criteria=u2 ~= 0  Threshold=0.5  InputSameDT=off
  phidr : Integrator  InitialCondition=phirdo
  phiqr : Integrator  InitialCondition=phirqo
  web : Gain  Gain=web  SaturateOnIntegerOverflow=on  OutDataTypeStr=Inherit: Same as input  ParamDataTypeStr=Inherit: Same as input
  web1 : Gain  Gain=web  SaturateOnIntegerOverflow=on  OutDataTypeStr=Inherit: Same as input  ParamDataTypeStr=Inherit: Same as input
  iqr,idr : Outport  VectorParamsAs1DForOutWhenUnconnected=off
  phiqr,phidr : Outport  Port=2  VectorParamsAs1DForOutWhenUnconnected=off
  wires:
  Mux3/1 -> phiqr,phidr/1
  Sum1/1 -> web1/1
  w-wr/1 -> Product/2, Product1/1
  Product/1 -> Sum2/2
  Sum2/1 -> web/1
  phidr/1 -> Switch2/3
  vqr,vdr/1 -> Demux/1
  Product1/1 -> Sum1/1
  Demux/2 -> Sum1/2
  1\Llr3/1 -> Sum1/3
  1\Llr2/1 -> 1\Llr3/1, Mux2/2  "idr"
  Sum4/1 -> 1\Llr2/1
  Demux1/2 -> Sum4/1
  Mux2/1 -> iqr,idr/1
  1\Llr/1 -> Mux2/1, 1\Llr1/1  "iqr"
  1\Llr1/1 -> Sum2/3
  Sum3/1 -> 1\Llr/1
  Demux/1 -> Sum2/1
  Demux1/1 -> Sum3/2
  phimq,phimd/1 -> Demux1/1
  web/1 -> Switch/3
  Switch/1 -> phiqr/1
  Constant/1 -> Switch/1, Switch1/1
  Switch1/1 -> Mux3/1, Product1/2, Sum3/1
  phiqr/1 -> Switch1/3  "phiqr"
  Switch2/1 -> Mux3/2, Sum4/2, Product/1
  Switch3/1 -> phidr/1
  web1/1 -> Switch3/3
  Constant1/1 -> Switch2/1, Switch3/1
  Trip/1 -> Switch/2, Switch3/2, Switch1/2, Switch2/2
